simulink model "PID"  (R2023a)
settings: Solver=VariableStepAuto  StartTime=0.0  StopTime=20  RelTol=1e-3
values from neighbouring files (symbols this model uses):
  b = Kb*e_reset*Ts    [PIDfunction.m]    (also in main.m = 0.16)
  Jm = 0.014    [main.m]
  Ke = 0.849    [main.m]
  Km = 0.849    [main.m]
  La = 1.71*10^-3    (= 0.00171)    [main.m]
  Ra = 0.327    [main.m]
  Ts = 0.01    [main.m]
settings Model: Creator=Admin  LastModifiedBy=admin
settings DebuggingCC: UnconnectedInputMsg=warning  UnconnectedOutputMsg=warning  UnconnectedLineMsg=warning
settings ModelReferenceCC: EnableRefExpFcnMdlSchedulingChecks=on
settings RTWCC: DLArmComputeVersion=19.05

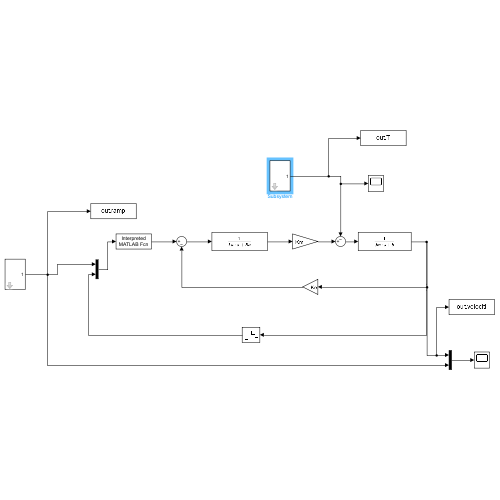
[thumbnail: Simulink's stored preview of the top-level diagram]
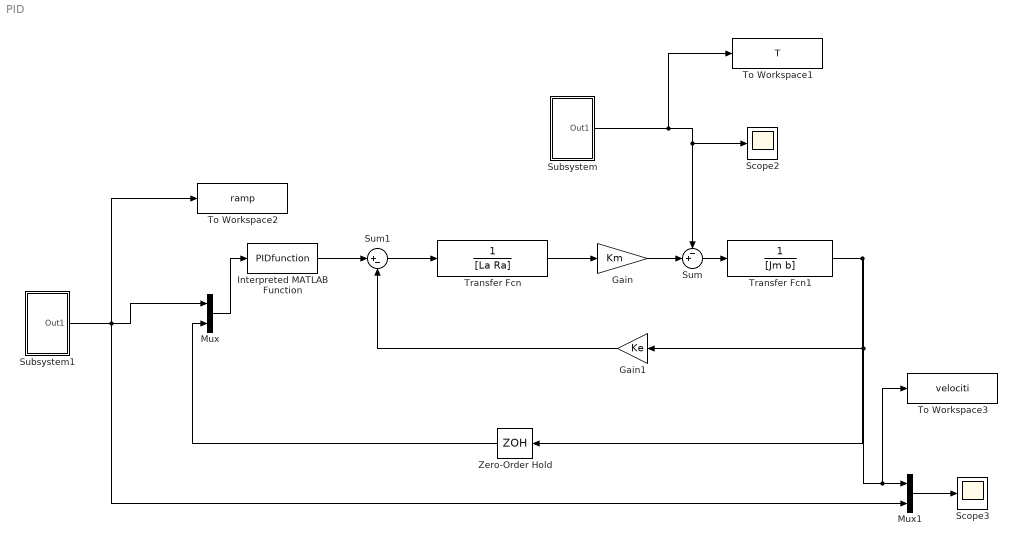
== system PID ==
  Gain : Gain  Gain=Km
  Gain1 : Gain  Gain=Ke
  Interpreted MATLAB Function : MATLABFcn  MATLABFcn=PIDfunction  OutputDimensions=1  OutputSignalType=real
  Mux : Mux  Inputs=2
  Mux1 : Mux  Inputs=2
  Scope2 : Scope
  Scope3 : Scope
  Subsystem : Subsystem  mask{t2=5, t1=3, a=5}
      mask prompts: t2 "stop_time"; t1 "start_time"; a "value"
  Subsystem1 : Subsystem  mask{t2=6, t1=0, a=24}
      mask prompts: t2 "stop_time"; t1 "start_time"; a "value"
  Sum : Sum  Inputs=-+|
  Sum1 : Sum  Inputs=|+-
  To Workspace1 : ToWorkspace  VariableName=T  SaveFormat=Timeseries  SampleTime=-1
  To Workspace2 : ToWorkspace  VariableName=ramp  SaveFormat=Timeseries  SampleTime=-1
  To Workspace3 : ToWorkspace  VariableName=velociti  SaveFormat=Timeseries  SampleTime=-1
  Transfer Fcn : TransferFcn  Denominator=[La Ra]
  Transfer Fcn1 : TransferFcn  Denominator=[Jm b]
  Zero-Order Hold : ZeroOrderHold  SampleTime=Ts
  wires:
  Transfer Fcn/1 -> Gain/1
  Sum/1 -> Transfer Fcn1/1
  Sum1/1 -> Transfer Fcn/1
  Gain1/1 -> Sum1/2
  Transfer Fcn1/1 -> Zero-Order Hold/1, To Workspace3/1, Mux1/1, Gain1/1
  Gain/1 -> Sum/2
  Zero-Order Hold/1 -> Mux/2
  Subsystem/1(Out1) -> Scope2/1, Sum/1, To Workspace1/1
  Subsystem1/1(Out1) -> To Workspace2/1, Mux1/2, Mux/1
  Mux1/1 -> Scope3/1
  Interpreted MATLAB Function/1 -> Sum1/1
  Mux/1 -> Interpreted MATLAB Function/1

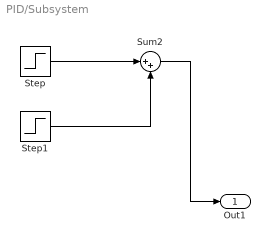
== system PID/Subsystem ==
  Step : Step  Time=t1  After=a  SampleTime=Ts
  Step1 : Step  Time=t2  After=-a  SampleTime=Ts
  Sum2 : Sum  Inputs=|++
  Out1 : Outport
  wires:
  Step/1 -> Sum2/1
  Step1/1 -> Sum2/2
  Sum2/1 -> Out1/1

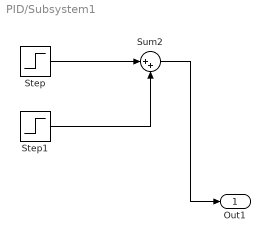
== system PID/Subsystem1 ==
  Step : Step  Time=t1  After=a  SampleTime=Ts
  Step1 : Step  Time=t2  After=-a  SampleTime=Ts
  Sum2 : Sum  Inputs=|++
  Out1 : Outport
  wires:
  Step/1 -> Sum2/1
  Step1/1 -> Sum2/2
  Sum2/1 -> Out1/1
